simulink model "ProcessNetworkSimulation"  (R2015b)
settings: Solver=VariableStepAuto  StartTime=0.0  StopTime=1000.0  RelTol=1e-3
libraries: simulink x1, simeventslib x1
(part 19 of 21)

== system ProcessNetworkSimulation/Process_48/Process ==
  OUTQueue : FIFOQueue  Capacity=inf
  ProcessQueue : FIFOQueue  Capacity=Inf  StatAverageWait=on  StatAverageQueueLength=on
      settings: OutputPortMap=o2,o3
  ProcessServer : NServer  NumberOfServers=13  ServiceTimeFrom=Signal port t  StatNumberDeparted=on  StatUtilization=on
      settings: OutputPortMap=o0,o5
  ProcessTime : EventBasedRandomNumber  meanExp=0.05  minUnif=1  meanNorm=2  stdNorm=0.2  Seed=7122
  Routing : EventBasedRandomNumber  Distribution=Arbitrary discrete  valueVecDisc=[0,1,2,3,4,5,6,7,8,9,10,11,12,13,14,15,16,17,18,19,20,21,22,23,24,25,26,27,28,29,30,31,32,33,34,35,36,37]  probVecDisc=[0,0.0093,0.0231,0.0139,0.0324,0.0324,0.0231,0.0231,0.0139,0.0459,0.0093,0.0093,0.0093,0.0463,0.0417,0.0417,0.0139,0.037,0.0417,0.0417,0.0324,0.0463,0.0463,0.0324,0.0093,0.0417,0.0093,0.0278,0.0278,0.0139,0.0417,0.0231,0.0093,0.0139,0.0324,0.0417,0.0417,0]  Seed=10339
  read_ProcessTimer : ReadTimer  TimerTag=T_Process_48  StatAverageTimeElapsed=on
      settings: OutputPortMap=o3
  setRouting : SetAttribute  AttributeName=outputFlowNode  AttributeFrom=Signal port  EvaluatedAttributeValue={ []}
  start_ProcessTimer : StartTimer  TimerTag=T_Process_48  TimerStartedOption=Restart
  IN_Job : PMIOPort  Port=1  Side=Left
  OUT_Job : PMIOPort  Port=2  Side=Right
  wires:
  Routing/1 -> setRouting/1
  ProcessTime/1 -> ProcessServer/1
  connections:
  setRouting/LConn1 -- OUTQueue/RConn1
  IN_Job/RConn1 -- start_ProcessTimer/LConn1
  ProcessServer/RConn1 -- read_ProcessTimer/LConn1
  start_ProcessTimer/RConn1 -- ProcessQueue/LConn1
  ProcessQueue/RConn1 -- ProcessServer/LConn1
  read_ProcessTimer/RConn1 -- OUTQueue/LConn1
  OUT_Job/RConn1 -- setRouting/RConn1

== system ProcessNetworkSimulation/Process_49/Process ==
  OUTQueue : FIFOQueue  Capacity=inf
  ProcessQueue : FIFOQueue  Capacity=Inf  StatAverageWait=on  StatAverageQueueLength=on
      settings: OutputPortMap=o2,o3
  ProcessServer : NServer  NumberOfServers=10  ServiceTimeFrom=Signal port t  StatNumberDeparted=on  StatUtilization=on
      settings: OutputPortMap=o0,o5
  ProcessTime : EventBasedRandomNumber  meanExp=0.05  minUnif=1  meanNorm=2  stdNorm=0.2  Seed=13556
  Routing : EventBasedRandomNumber  Distribution=Arbitrary discrete  valueVecDisc=[0,1,2,3,4,5,6,7,8,9,10,11,12,13,14,15,16,17,18,19,20,21,22,23,24,25,26,27,28,29,30,31,32,33,34,35,36,37,38,39,40]  probVecDisc=[0,0.026,0.0104,0.0052,0.026,0.0104,0.0313,0.0104,0.0156,0.0467,0.026,0.0052,0.0104,0.0104,0.0469,0.0156,0.0469,0.0469,0.0104,0.0156,0.0104,0.0365,0.0469,0.0052,0.0156,0.0313,0.0313,0.0365,0.0156,0.0313,0.0365,0.0469,0.0313,0.0156,0.0469,0.0313,0.0156,0.0417,0.0469,0.0104,0]  Seed=16773
  read_ProcessTimer : ReadTimer  TimerTag=T_Process_49  StatAverageTimeElapsed=on
      settings: OutputPortMap=o3
  setRouting : SetAttribute  AttributeName=outputFlowNode  AttributeFrom=Signal port  EvaluatedAttributeValue={ []}
  start_ProcessTimer : StartTimer  TimerTag=T_Process_49  TimerStartedOption=Restart
  IN_Job : PMIOPort  Port=1  Side=Left
  OUT_Job : PMIOPort  Port=2  Side=Right
  wires:
  Routing/1 -> setRouting/1
  ProcessTime/1 -> ProcessServer/1
  connections:
  setRouting/LConn1 -- OUTQueue/RConn1
  IN_Job/RConn1 -- start_ProcessTimer/LConn1
  ProcessServer/RConn1 -- read_ProcessTimer/LConn1
  start_ProcessTimer/RConn1 -- ProcessQueue/LConn1
  ProcessQueue/RConn1 -- ProcessServer/LConn1
  read_ProcessTimer/RConn1 -- OUTQueue/LConn1
  OUT_Job/RConn1 -- setRouting/RConn1

== system ProcessNetworkSimulation/Process_5/Process ==
  OUTQueue : FIFOQueue  Capacity=inf
  ProcessQueue : FIFOQueue  Capacity=Inf  StatAverageWait=on  StatAverageQueueLength=on
      settings: OutputPortMap=o2,o3
  ProcessServer : NServer  NumberOfServers=9  ServiceTimeFrom=Signal port t  StatNumberDeparted=on  StatUtilization=on
      settings: OutputPortMap=o0,o5
  ProcessTime : EventBasedRandomNumber  meanExp=0.05  minUnif=1  meanNorm=2  stdNorm=0.2  Seed=19990
  Routing : EventBasedRandomNumber  Distribution=Arbitrary discrete  valueVecDisc=[0,1,2,3,4,5,6,7,8,9,10,11,12,13,14,15,16,17,18,19,20,21,22,23,24,25,26,27,28,29,30,31,32,33,34,35,36]  probVecDisc=[0,0.0337,0.0112,0.0506,0.0337,0.0056,0.0506,0.0506,0.0112,0.0281,0.0112,0.0281,0.0506,0.0506,0.0112,0.0112,0.0169,0.0393,0.0393,0.0393,0.0112,0.0112,0.0112,0.0112,0.0393,0.0112,0.0506,0.0565,0.0337,0.0281,0.0112,0.0112,0.0112,0.0449,0.0337,0.0506,0]  Seed=23207
  read_ProcessTimer : ReadTimer  TimerTag=T_Process_5  StatAverageTimeElapsed=on
      settings: OutputPortMap=o3
  setRouting : SetAttribute  AttributeName=outputFlowNode  AttributeFrom=Signal port  EvaluatedAttributeValue={ []}
  start_ProcessTimer : StartTimer  TimerTag=T_Process_5  TimerStartedOption=Restart
  IN_Job : PMIOPort  Port=1  Side=Left
  OUT_Job : PMIOPort  Port=2  Side=Right
  wires:
  Routing/1 -> setRouting/1
  ProcessTime/1 -> ProcessServer/1
  connections:
  setRouting/LConn1 -- OUTQueue/RConn1
  IN_Job/RConn1 -- start_ProcessTimer/LConn1
  ProcessServer/RConn1 -- read_ProcessTimer/LConn1
  start_ProcessTimer/RConn1 -- ProcessQueue/LConn1
  ProcessQueue/RConn1 -- ProcessServer/LConn1
  read_ProcessTimer/RConn1 -- OUTQueue/LConn1
  OUT_Job/RConn1 -- setRouting/RConn1

== system ProcessNetworkSimulation/Process_50/Process ==
  OUTQueue : FIFOQueue  Capacity=inf
  ProcessQueue : FIFOQueue  Capacity=Inf  StatAverageWait=on  StatAverageQueueLength=on
      settings: OutputPortMap=o2,o3
  ProcessServer : NServer  NumberOfServers=14  ServiceTimeFrom=Signal port t  StatNumberDeparted=on  StatUtilization=on
      settings: OutputPortMap=o0,o5
  ProcessTime : EventBasedRandomNumber  meanExp=0.05  minUnif=1  meanNorm=2  stdNorm=0.2  Seed=26424
  Routing : EventBasedRandomNumber  Distribution=Arbitrary discrete  valueVecDisc=[0,1,2,3,4,5,6,7,8,9,10,11,12,13,14,15,16,17,18,19,20,21,22,23,24,25,26,27,28,29,30,31,32,33,34,35,36,37,38,39,40,41]  probVecDisc=[0,0.0207,0.0207,0.0331,0.0372,0.0289,0.0124,0.0372,0.0289,0.0207,0.0124,0.0083,0.0248,0.0289,0.0372,0.0083,0.0372,0.0372,0.0083,0.0124,0.0372,0.0083,0.0372,0.0207,0.0289,0.0289,0.0289,0.0207,0.0331,0.0248,0.0372,0.0248,0.0083,0.0408,0.0372,0.0248,0.0372,0.0207,0.0124,0.0083,0.0248,0]  Seed=29641
  read_ProcessTimer : ReadTimer  TimerTag=T_Process_50  StatAverageTimeElapsed=on
      settings: OutputPortMap=o3
  setRouting : SetAttribute  AttributeName=outputFlowNode  AttributeFrom=Signal port  EvaluatedAttributeValue={ []}
  start_ProcessTimer : StartTimer  TimerTag=T_Process_50  TimerStartedOption=Restart
  IN_Job : PMIOPort  Port=1  Side=Left
  OUT_Job : PMIOPort  Port=2  Side=Right
  wires:
  Routing/1 -> setRouting/1
  ProcessTime/1 -> ProcessServer/1
  connections:
  setRouting/LConn1 -- OUTQueue/RConn1
  IN_Job/RConn1 -- start_ProcessTimer/LConn1
  ProcessServer/RConn1 -- read_ProcessTimer/LConn1
  start_ProcessTimer/RConn1 -- ProcessQueue/LConn1
  ProcessQueue/RConn1 -- ProcessServer/LConn1
  read_ProcessTimer/RConn1 -- OUTQueue/LConn1
  OUT_Job/RConn1 -- setRouting/RConn1

== system ProcessNetworkSimulation/Process_51/Process ==
  OUTQueue : FIFOQueue  Capacity=inf
  ProcessQueue : FIFOQueue  Capacity=Inf  StatAverageWait=on  StatAverageQueueLength=on
      settings: OutputPortMap=o2,o3
  ProcessServer : NServer  NumberOfServers=12  ServiceTimeFrom=Signal port t  StatNumberDeparted=on  StatUtilization=on
      settings: OutputPortMap=o0,o5
  ProcessTime : EventBasedRandomNumber  meanExp=0.05  minUnif=1  meanNorm=2  stdNorm=0.2  Seed=32858
  Routing : EventBasedRandomNumber  Distribution=Arbitrary discrete  valueVecDisc=[0,1,2,3,4,5,6,7,8,9,10,11,12,13,14,15,16,17,18,19,20,21,22,23,24,25,26,27,28,29,30,31,32,33,34,35,36,37,38]  probVecDisc=[0,0.0506,0.0462,0.0308,0.0359,0.0308,0.0256,0.0359,0.0308,0.0359,0.0154,0.0359,0.0256,0.0103,0.0256,0.0154,0.0308,0.0103,0.0513,0.0103,0.0359,0.0103,0.0154,0.0103,0.0359,0.0103,0.0154,0.0103,0.0103,0.041,0.0308,0.0103,0.0462,0.0462,0.0359,0.0462,0.0103,0.0256,0]  Seed=36075
  read_ProcessTimer : ReadTimer  TimerTag=T_Process_51  StatAverageTimeElapsed=on
      settings: OutputPortMap=o3
  setRouting : SetAttribute  AttributeName=outputFlowNode  AttributeFrom=Signal port  EvaluatedAttributeValue={ []}
  start_ProcessTimer : StartTimer  TimerTag=T_Process_51  TimerStartedOption=Restart
  IN_Job : PMIOPort  Port=1  Side=Left
  OUT_Job : PMIOPort  Port=2  Side=Right
  wires:
  Routing/1 -> setRouting/1
  ProcessTime/1 -> ProcessServer/1
  connections:
  setRouting/LConn1 -- OUTQueue/RConn1
  IN_Job/RConn1 -- start_ProcessTimer/LConn1
  ProcessServer/RConn1 -- read_ProcessTimer/LConn1
  start_ProcessTimer/RConn1 -- ProcessQueue/LConn1
  ProcessQueue/RConn1 -- ProcessServer/LConn1
  read_ProcessTimer/RConn1 -- OUTQueue/LConn1
  OUT_Job/RConn1 -- setRouting/RConn1

== system ProcessNetworkSimulation/Process_52/Process ==
  OUTQueue : FIFOQueue  Capacity=inf
  ProcessQueue : FIFOQueue  Capacity=Inf  StatAverageWait=on  StatAverageQueueLength=on
      settings: OutputPortMap=o2,o3
  ProcessServer : NServer  NumberOfServers=12  ServiceTimeFrom=Signal port t  StatNumberDeparted=on  StatUtilization=on
      settings: OutputPortMap=o0,o5
  ProcessTime : EventBasedRandomNumber  meanExp=0.05  minUnif=1  meanNorm=2  stdNorm=0.2  Seed=39292
  Routing : EventBasedRandomNumber  Distribution=Arbitrary discrete  valueVecDisc=[0,1,2,3,4,5,6,7,8,9,10,11,12,13,14,15,16,17,18,19,20,21,22,23,24,25,26,27,28,29,30,31,32,33,34,35]  probVecDisc=[0,0.0428,0.0481,0.0107,0.0428,0.0481,0.0107,0.0481,0.0267,0.0481,0.0374,0.0481,0.016,0.0267,0.016,0.0481,0.0053,0.0107,0.0541,0.0321,0.016,0.0321,0.0374,0.0535,0.0267,0.0053,0.016,0.0374,0.0107,0.0481,0.0374,0.0321,0.0053,0.0107,0.0107,0]  Seed=42508
  read_ProcessTimer : ReadTimer  TimerTag=T_Process_52  StatAverageTimeElapsed=on
      settings: OutputPortMap=o3
  setRouting : SetAttribute  AttributeName=outputFlowNode  AttributeFrom=Signal port  EvaluatedAttributeValue={ []}
  start_ProcessTimer : StartTimer  TimerTag=T_Process_52  TimerStartedOption=Restart
  IN_Job : PMIOPort  Port=1  Side=Left
  OUT_Job : PMIOPort  Port=2  Side=Right
  wires:
  Routing/1 -> setRouting/1
  ProcessTime/1 -> ProcessServer/1
  connections:
  setRouting/LConn1 -- OUTQueue/RConn1
  IN_Job/RConn1 -- start_ProcessTimer/LConn1
  ProcessServer/RConn1 -- read_ProcessTimer/LConn1
  start_ProcessTimer/RConn1 -- ProcessQueue/LConn1
  ProcessQueue/RConn1 -- ProcessServer/LConn1
  read_ProcessTimer/RConn1 -- OUTQueue/LConn1
  OUT_Job/RConn1 -- setRouting/RConn1

== system ProcessNetworkSimulation/Process_53/Process ==
  OUTQueue : FIFOQueue  Capacity=inf
  ProcessQueue : FIFOQueue  Capacity=Inf  StatAverageWait=on  StatAverageQueueLength=on
      settings: OutputPortMap=o2,o3
  ProcessServer : NServer  NumberOfServers=10  ServiceTimeFrom=Signal port t  StatNumberDeparted=on  StatUtilization=on
      settings: OutputPortMap=o0,o5
  ProcessTime : EventBasedRandomNumber  meanExp=0.05  minUnif=1  meanNorm=2  stdNorm=0.2  Seed=45725
  Routing : EventBasedRandomNumber  Distribution=Arbitrary discrete  valueVecDisc=[0,1,2,3,4,5,6,7,8,9,10,11,12,13,14,15,16,17,18,19,20,21,22,23,24,25,26,27,28,29,30,31,32,33,34,35,36,37,38,39]  probVecDisc=[0,0.0433,0.024,0.0096,0.0482,0.0096,0.0144,0.0288,0.0433,0.0096,0.0144,0.0337,0.0096,0.024,0.0144,0.0096,0.0288,0.0096,0.0288,0.0096,0.024,0.0433,0.024,0.024,0.0144,0.0433,0.0096,0.0096,0.0433,0.0337,0.0385,0.0096,0.0096,0.0481,0.0433,0.0481,0.0433,0.0433,0.0337,0]  Seed=48942
  read_ProcessTimer : ReadTimer  TimerTag=T_Process_53  StatAverageTimeElapsed=on
      settings: OutputPortMap=o3
  setRouting : SetAttribute  AttributeName=outputFlowNode  AttributeFrom=Signal port  EvaluatedAttributeValue={ []}
  start_ProcessTimer : StartTimer  TimerTag=T_Process_53  TimerStartedOption=Restart
  IN_Job : PMIOPort  Port=1  Side=Left
  OUT_Job : PMIOPort  Port=2  Side=Right
  wires:
  Routing/1 -> setRouting/1
  ProcessTime/1 -> ProcessServer/1
  connections:
  setRouting/LConn1 -- OUTQueue/RConn1
  IN_Job/RConn1 -- start_ProcessTimer/LConn1
  ProcessServer/RConn1 -- read_ProcessTimer/LConn1
  start_ProcessTimer/RConn1 -- ProcessQueue/LConn1
  ProcessQueue/RConn1 -- ProcessServer/LConn1
  read_ProcessTimer/RConn1 -- OUTQueue/LConn1
  OUT_Job/RConn1 -- setRouting/RConn1

== system ProcessNetworkSimulation/Process_54/Process ==
  OUTQueue : FIFOQueue  Capacity=inf
  ProcessQueue : FIFOQueue  Capacity=Inf  StatAverageWait=on  StatAverageQueueLength=on
      settings: OutputPortMap=o2,o3
  ProcessServer : NServer  NumberOfServers=11  ServiceTimeFrom=Signal port t  StatNumberDeparted=on  StatUtilization=on
      settings: OutputPortMap=o0,o5
  ProcessTime : EventBasedRandomNumber  meanExp=0.05  minUnif=1  meanNorm=2  stdNorm=0.2  Seed=52159
  Routing : EventBasedRandomNumber  Distribution=Arbitrary discrete  valueVecDisc=[0,1,2,3,4,5,6,7,8,9,10,11,12,13,14,15,16,17,18,19,20,21,22,23,24,25,26,27,28,29,30,31,32,33,34,35,36,37,38,39,40,41,42,43,44,45,46,47,48,49,50,51]  probVecDisc=[0,0.0174,0.0313,0.0104,0.0278,0.0104,0.0069,0.0035,0.0069,0.0346,0.0208,0.0069,0.0069,0.0347,0.0069,0.0313,0.0278,0.0174,0.0035,0.0243,0.0069,0.0313,0.0069,0.0313,0.0313,0.0208,0.0243,0.0243,0.0243,0.0104,0.0243,0.0243,0.0313,0.0243,0.0174,0.0313,0.0174,0.0069,0.0243,0.0104,0.0208,0.0313,0.0174,0.0313,0.0243,0.0278,0.0208,0.0104,0.0208,0.0104,0.0313,0]  Seed=55376
  read_ProcessTimer : ReadTimer  TimerTag=T_Process_54  StatAverageTimeElapsed=on
      settings: OutputPortMap=o3
  setRouting : SetAttribute  AttributeName=outputFlowNode  AttributeFrom=Signal port  EvaluatedAttributeValue={ []}
  start_ProcessTimer : StartTimer  TimerTag=T_Process_54  TimerStartedOption=Restart
  IN_Job : PMIOPort  Port=1  Side=Left
  OUT_Job : PMIOPort  Port=2  Side=Right
  wires:
  Routing/1 -> setRouting/1
  ProcessTime/1 -> ProcessServer/1
  connections:
  setRouting/LConn1 -- OUTQueue/RConn1
  IN_Job/RConn1 -- start_ProcessTimer/LConn1
  ProcessServer/RConn1 -- read_ProcessTimer/LConn1
  start_ProcessTimer/RConn1 -- ProcessQueue/LConn1
  ProcessQueue/RConn1 -- ProcessServer/LConn1
  read_ProcessTimer/RConn1 -- OUTQueue/LConn1
  OUT_Job/RConn1 -- setRouting/RConn1

== system ProcessNetworkSimulation/Process_55/Process ==
  OUTQueue : FIFOQueue  Capacity=inf
  ProcessQueue : FIFOQueue  Capacity=Inf  StatAverageWait=on  StatAverageQueueLength=on
      settings: OutputPortMap=o2,o3
  ProcessServer : NServer  NumberOfServers=13  ServiceTimeFrom=Signal port t  StatNumberDeparted=on  StatUtilization=on
      settings: OutputPortMap=o0,o5
  ProcessTime : EventBasedRandomNumber  meanExp=0.05  minUnif=1  meanNorm=2  stdNorm=0.2  Seed=58593
  Routing : EventBasedRandomNumber  Distribution=Arbitrary discrete  valueVecDisc=[0,1,2,3,4,5,6,7,8,9,10,11,12,13,14,15,16,17,18,19,20,21,22,23,24,25,26,27,28,29,30,31,32,33,34,35,36,37,38,39,40,41,42,43,44,45,46]  probVecDisc=[0,0.0297,0.0381,0.0339,0.0381,0.0085,0.0381,0.0381,0.0127,0.0085,0.0085,0.0339,0.0254,0.0042,0.0085,0.0085,0.0297,0.0127,0.0085,0.0085,0.0421,0.0297,0.0212,0.0424,0.0212,0.0424,0.0085,0.0381,0.0297,0.0085,0.0297,0.0127,0.0297,0.0042,0.0127,0.0212,0.0254,0.0085,0.0297,0.0254,0.0042,0.0297,0.0085,0.0042,0.0127,0.0424,0.0212]  Seed=61810
  read_ProcessTimer : ReadTimer  TimerTag=T_Process_55  StatAverageTimeElapsed=on
      settings: OutputPortMap=o3
  setRouting : SetAttribute  AttributeName=outputFlowNode  AttributeFrom=Signal port  EvaluatedAttributeValue={ []}
  start_ProcessTimer : StartTimer  TimerTag=T_Process_55  TimerStartedOption=Restart
  IN_Job : PMIOPort  Port=1  Side=Left
  OUT_Job : PMIOPort  Port=2  Side=Right
  wires:
  Routing/1 -> setRouting/1
  ProcessTime/1 -> ProcessServer/1
  connections:
  setRouting/LConn1 -- OUTQueue/RConn1
  IN_Job/RConn1 -- start_ProcessTimer/LConn1
  ProcessServer/RConn1 -- read_ProcessTimer/LConn1
  start_ProcessTimer/RConn1 -- ProcessQueue/LConn1
  ProcessQueue/RConn1 -- ProcessServer/LConn1
  read_ProcessTimer/RConn1 -- OUTQueue/LConn1
  OUT_Job/RConn1 -- setRouting/RConn1

== system ProcessNetworkSimulation/Process_56/Process ==
  OUTQueue : FIFOQueue  Capacity=inf
  ProcessQueue : FIFOQueue  Capacity=Inf  StatAverageWait=on  StatAverageQueueLength=on
      settings: OutputPortMap=o2,o3
  ProcessServer : NServer  NumberOfServers=11  ServiceTimeFrom=Signal port t  StatNumberDeparted=on  StatUtilization=on
      settings: OutputPortMap=o0,o5
  ProcessTime : EventBasedRandomNumber  meanExp=0.05  minUnif=1  meanNorm=2  stdNorm=0.2  Seed=65027
  Routing : EventBasedRandomNumber  Distribution=Arbitrary discrete  valueVecDisc=[0,1,2,3,4,5,6,7,8,9,10,11,12,13,14,15,16,17,18,19,20,21,22,23,24,25,26,27,28,29,30,31,32,33,34,35,36,37,38,39]  probVecDisc=[0,0.0097,0.0242,0.0338,0.0429,0.0097,0.0386,0.0338,0.029,0.0338,0.0145,0.0435,0.029,0.0097,0.0338,0.0242,0.0435,0.0435,0.0435,0.0338,0.0435,0.0242,0.0338,0.0097,0.0435,0.0097,0.0145,0.0145,0.0145,0.029,0.0097,0.0338,0.0435,0.0097,0.0338,0.0097,0.0097,0.0097,0.029,0]  Seed=2708
  read_ProcessTimer : ReadTimer  TimerTag=T_Process_56  StatAverageTimeElapsed=on
      settings: OutputPortMap=o3
  setRouting : SetAttribute  AttributeName=outputFlowNode  AttributeFrom=Signal port  EvaluatedAttributeValue={ []}
  start_ProcessTimer : StartTimer  TimerTag=T_Process_56  TimerStartedOption=Restart
  IN_Job : PMIOPort  Port=1  Side=Left
  OUT_Job : PMIOPort  Port=2  Side=Right
  wires:
  Routing/1 -> setRouting/1
  ProcessTime/1 -> ProcessServer/1
  connections:
  setRouting/LConn1 -- OUTQueue/RConn1
  IN_Job/RConn1 -- start_ProcessTimer/LConn1
  ProcessServer/RConn1 -- read_ProcessTimer/LConn1
  start_ProcessTimer/RConn1 -- ProcessQueue/LConn1
  ProcessQueue/RConn1 -- ProcessServer/LConn1
  read_ProcessTimer/RConn1 -- OUTQueue/LConn1
  OUT_Job/RConn1 -- setRouting/RConn1

== system ProcessNetworkSimulation/Process_57/Process ==
  OUTQueue : FIFOQueue  Capacity=inf
  ProcessQueue : FIFOQueue  Capacity=Inf  StatAverageWait=on  StatAverageQueueLength=on
      settings: OutputPortMap=o2,o3
  ProcessServer : NServer  NumberOfServers=10  ServiceTimeFrom=Signal port t  StatNumberDeparted=on  StatUtilization=on
      settings: OutputPortMap=o0,o5
  ProcessTime : EventBasedRandomNumber  meanExp=0.05  minUnif=1  meanNorm=2  stdNorm=0.2  Seed=5925
  Routing : EventBasedRandomNumber  Distribution=Arbitrary discrete  valueVecDisc=[0,1,2,3,4,5,6,7,8,9,10,11,12,13,14,15,16,17,18,19,20,21,22,23,24,25,26,27,28,29,30,31,32]  probVecDisc=[0,0.0353,0.0118,0.0294,0.0118,0.0471,0.0527,0.0529,0.0471,0.0294,0.0176,0.0529,0.0353,0.0353,0.0353,0.0353,0.0353,0.0294,0.0412,0.0353,0.0412,0.0412,0.0118,0.0294,0.0118,0.0353,0.0412,0.0118,0.0118,0.0353,0.0412,0.0176,0]  Seed=9142
  read_ProcessTimer : ReadTimer  TimerTag=T_Process_57  StatAverageTimeElapsed=on
      settings: OutputPortMap=o3
  setRouting : SetAttribute  AttributeName=outputFlowNode  AttributeFrom=Signal port  EvaluatedAttributeValue={ []}
  start_ProcessTimer : StartTimer  TimerTag=T_Process_57  TimerStartedOption=Restart
  IN_Job : PMIOPort  Port=1  Side=Left
  OUT_Job : PMIOPort  Port=2  Side=Right
  wires:
  Routing/1 -> setRouting/1
  ProcessTime/1 -> ProcessServer/1
  connections:
  setRouting/LConn1 -- OUTQueue/RConn1
  IN_Job/RConn1 -- start_ProcessTimer/LConn1
  ProcessServer/RConn1 -- read_ProcessTimer/LConn1
  start_ProcessTimer/RConn1 -- ProcessQueue/LConn1
  ProcessQueue/RConn1 -- ProcessServer/LConn1
  read_ProcessTimer/RConn1 -- OUTQueue/LConn1
  OUT_Job/RConn1 -- setRouting/RConn1

== system ProcessNetworkSimulation/Process_58/Process ==
  OUTQueue : FIFOQueue  Capacity=inf
  ProcessQueue : FIFOQueue  Capacity=Inf  StatAverageWait=on  StatAverageQueueLength=on
      settings: OutputPortMap=o2,o3
  ProcessServer : NServer  NumberOfServers=15  ServiceTimeFrom=Signal port t  StatNumberDeparted=on  StatUtilization=on
      settings: OutputPortMap=o0,o5
  ProcessTime : EventBasedRandomNumber  meanExp=0.05  minUnif=1  meanNorm=2  stdNorm=0.2  Seed=12359
  Routing : EventBasedRandomNumber  Distribution=Arbitrary discrete  valueVecDisc=[0,1,2,3,4,5,6,7,8,9,10,11,12,13,14,15,16,17,18,19,20,21,22,23,24,25,26,27,28,29,30,31,32,33,34,35,36,37,38,39,40,41,42,43]  probVecDisc=[0,0.0345,0.0307,0.0345,0.0268,0.0192,0.0115,0.0192,0.023,0.0345,0.0077,0.0345,0.0192,0.0115,0.023,0.023,0.023,0.023,0.0038,0.0345,0.023,0.0307,0.0345,0.023,0.0192,0.0192,0.023,0.0115,0.0268,0.0268,0.0038,0.0345,0.0268,0.0345,0.0115,0.0115,0.0378,0.0268,0.0345,0.0307,0.0345,0.0115,0.0268,0]  Seed=15576
  read_ProcessTimer : ReadTimer  TimerTag=T_Process_58  StatAverageTimeElapsed=on
      settings: OutputPortMap=o3
  setRouting : SetAttribute  AttributeName=outputFlowNode  AttributeFrom=Signal port  EvaluatedAttributeValue={ []}
  start_ProcessTimer : StartTimer  TimerTag=T_Process_58  TimerStartedOption=Restart
  IN_Job : PMIOPort  Port=1  Side=Left
  OUT_Job : PMIOPort  Port=2  Side=Right
  wires:
  Routing/1 -> setRouting/1
  ProcessTime/1 -> ProcessServer/1
  connections:
  setRouting/LConn1 -- OUTQueue/RConn1
  IN_Job/RConn1 -- start_ProcessTimer/LConn1
  ProcessServer/RConn1 -- read_ProcessTimer/LConn1
  start_ProcessTimer/RConn1 -- ProcessQueue/LConn1
  ProcessQueue/RConn1 -- ProcessServer/LConn1
  read_ProcessTimer/RConn1 -- OUTQueue/LConn1
  OUT_Job/RConn1 -- setRouting/RConn1

== system ProcessNetworkSimulation/Process_59/Process ==
  OUTQueue : FIFOQueue  Capacity=inf
  ProcessQueue : FIFOQueue  Capacity=Inf  StatAverageWait=on  StatAverageQueueLength=on
      settings: OutputPortMap=o2,o3
  ProcessServer : NServer  NumberOfServers=14  ServiceTimeFrom=Signal port t  StatNumberDeparted=on  StatUtilization=on
      settings: OutputPortMap=o0,o5
  ProcessTime : EventBasedRandomNumber  meanExp=0.05  minUnif=1  meanNorm=2  stdNorm=0.2  Seed=18793
  Routing : EventBasedRandomNumber  Distribution=Arbitrary discrete  valueVecDisc=[0,1,2,3,4,5,6,7,8,9,10,11,12,13,14,15,16,17,18,19,20,21,22,23,24,25,26,27,28,29,30,31,32,33,34,35,36,37,38,39,40,41,42,43,44]  probVecDisc=[0,0.009,0.009,0.009,0.027,0.0045,0.009,0.036,0.0225,0.0315,0.0225,0.0045,0.009,0.009,0.0405,0.0135,0.009,0.0405,0.027,0.0225,0.0315,0.027,0.0315,0.0135,0.0405,0.036,0.027,0.0405,0.027,0.0045,0.0315,0.0315,0.009,0.046,0.0135,0.009,0.0225,0.045,0.009,0.0405,0.009,0.027,0.0405,0.0315,0]  Seed=22010
  read_ProcessTimer : ReadTimer  TimerTag=T_Process_59  StatAverageTimeElapsed=on
      settings: OutputPortMap=o3
  setRouting : SetAttribute  AttributeName=outputFlowNode  AttributeFrom=Signal port  EvaluatedAttributeValue={ []}
  start_ProcessTimer : StartTimer  TimerTag=T_Process_59  TimerStartedOption=Restart
  IN_Job : PMIOPort  Port=1  Side=Left
  OUT_Job : PMIOPort  Port=2  Side=Right
  wires:
  Routing/1 -> setRouting/1
  ProcessTime/1 -> ProcessServer/1
  connections:
  setRouting/LConn1 -- OUTQueue/RConn1
  IN_Job/RConn1 -- start_ProcessTimer/LConn1
  ProcessServer/RConn1 -- read_ProcessTimer/LConn1
  start_ProcessTimer/RConn1 -- ProcessQueue/LConn1
  ProcessQueue/RConn1 -- ProcessServer/LConn1
  read_ProcessTimer/RConn1 -- OUTQueue/LConn1
  OUT_Job/RConn1 -- setRouting/RConn1

== system ProcessNetworkSimulation/Process_6/Process ==
  OUTQueue : FIFOQueue  Capacity=inf
  ProcessQueue : FIFOQueue  Capacity=Inf  StatAverageWait=on  StatAverageQueueLength=on
      settings: OutputPortMap=o2,o3
  ProcessServer : NServer  NumberOfServers=13  ServiceTimeFrom=Signal port t  StatNumberDeparted=on  StatUtilization=on
      settings: OutputPortMap=o0,o5
  ProcessTime : EventBasedRandomNumber  meanExp=0.05  minUnif=1  meanNorm=2  stdNorm=0.2  Seed=25227
  Routing : EventBasedRandomNumber  Distribution=Arbitrary discrete  valueVecDisc=[0,1,2,3,4,5,6,7,8,9,10,11,12,13,14,15,16,17,18,19,20,21,22,23,24,25,26,27,28,29,30,31,32,33,34,35,36,37,38,39]  probVecDisc=[0,0.0096,0.0433,0.0337,0.0433,0.0337,0.0433,0.0337,0.0385,0.0288,0.0433,0.0433,0.024,0.0288,0.0144,0.0096,0.0433,0.0288,0.0433,0.0433,0.0482,0.0144,0.0144,0.0288,0.0433,0.0288,0.0096,0.0096,0.0144,0.0096,0.0096,0.0096,0.0096,0.0385,0.0048,0.0144,0.0096,0.0288,0.0144,0.0096]  Seed=28444
  read_ProcessTimer : ReadTimer  TimerTag=T_Process_6  StatAverageTimeElapsed=on
      settings: OutputPortMap=o3
  setRouting : SetAttribute  AttributeName=outputFlowNode  AttributeFrom=Signal port  EvaluatedAttributeValue={ []}
  start_ProcessTimer : StartTimer  TimerTag=T_Process_6  TimerStartedOption=Restart
  IN_Job : PMIOPort  Port=1  Side=Left
  OUT_Job : PMIOPort  Port=2  Side=Right
  wires:
  Routing/1 -> setRouting/1
  ProcessTime/1 -> ProcessServer/1
  connections:
  setRouting/LConn1 -- OUTQueue/RConn1
  IN_Job/RConn1 -- start_ProcessTimer/LConn1
  ProcessServer/RConn1 -- read_ProcessTimer/LConn1
  start_ProcessTimer/RConn1 -- ProcessQueue/LConn1
  ProcessQueue/RConn1 -- ProcessServer/LConn1
  read_ProcessTimer/RConn1 -- OUTQueue/LConn1
  OUT_Job/RConn1 -- setRouting/RConn1

== system ProcessNetworkSimulation/Process_60/Process ==
  OUTQueue : FIFOQueue  Capacity=inf
  ProcessQueue : FIFOQueue  Capacity=Inf  StatAverageWait=on  StatAverageQueueLength=on
      settings: OutputPortMap=o2,o3
  ProcessServer : NServer  NumberOfServers=11  ServiceTimeFrom=Signal port t  StatNumberDeparted=on  StatUtilization=on
      settings: OutputPortMap=o0,o5
  ProcessTime : EventBasedRandomNumber  meanExp=0.05  minUnif=1  meanNorm=2  stdNorm=0.2  Seed=31661
  Routing : EventBasedRandomNumber  Distribution=Arbitrary discrete  valueVecDisc=[0,1,2,3,4,5,6,7,8,9,10,11,12,13,14,15,16,17,18,19,20,21,22,23,24,25,26,27,28,29,30,31,32,33,34,35,36,37,38,39,40,41]  probVecDisc=[0,0.0424,0.0378,0.0126,0.0378,0.0294,0.0378,0.021,0.0378,0.0336,0.0084,0.0252,0.0378,0.042,0.0042,0.0252,0.021,0.0084,0.0126,0.0294,0.0294,0.0294,0.0336,0.0126,0.021,0.0378,0.0252,0.0084,0.0252,0.0378,0.0084,0.0084,0.0378,0.0378,0.0294,0.0294,0.0084,0.0126,0.0126,0.021,0.0294,0]  Seed=34878
  read_ProcessTimer : ReadTimer  TimerTag=T_Process_60  StatAverageTimeElapsed=on
      settings: OutputPortMap=o3
  setRouting : SetAttribute  AttributeName=outputFlowNode  AttributeFrom=Signal port  EvaluatedAttributeValue={ []}
  start_ProcessTimer : StartTimer  TimerTag=T_Process_60  TimerStartedOption=Restart
  IN_Job : PMIOPort  Port=1  Side=Left
  OUT_Job : PMIOPort  Port=2  Side=Right
  wires:
  Routing/1 -> setRouting/1
  ProcessTime/1 -> ProcessServer/1
  connections:
  setRouting/LConn1 -- OUTQueue/RConn1
  IN_Job/RConn1 -- start_ProcessTimer/LConn1
  ProcessServer/RConn1 -- read_ProcessTimer/LConn1
  start_ProcessTimer/RConn1 -- ProcessQueue/LConn1
  ProcessQueue/RConn1 -- ProcessServer/LConn1
  read_ProcessTimer/RConn1 -- OUTQueue/LConn1
  OUT_Job/RConn1 -- setRouting/RConn1

== system ProcessNetworkSimulation/Process_61/Process ==
  OUTQueue : FIFOQueue  Capacity=inf
  ProcessQueue : FIFOQueue  Capacity=Inf  StatAverageWait=on  StatAverageQueueLength=on
      settings: OutputPortMap=o2,o3
  ProcessServer : NServer  NumberOfServers=14  ServiceTimeFrom=Signal port t  StatNumberDeparted=on  StatUtilization=on
      settings: OutputPortMap=o0,o5
  ProcessTime : EventBasedRandomNumber  meanExp=0.05  minUnif=1  meanNorm=2  stdNorm=0.2  Seed=38095
  Routing : EventBasedRandomNumber  Distribution=Arbitrary discrete  valueVecDisc=[0,1,2,3,4,5,6,7,8,9,10,11,12,13,14,15,16,17,18,19,20,21,22,23,24,25,26,27,28,29,30,31,32,33,34,35,36,37,38,39,40,41,42,43,44]  probVecDisc=[0,0.0039,0.0349,0.038,0.0271,0.0078,0.0349,0.0349,0.0349,0.0349,0.0078,0.0078,0.0116,0.0233,0.0116,0.0271,0.0078,0.0349,0.0349,0.0194,0.0388,0.0078,0.0194,0.0078,0.0233,0.0078,0.0349,0.0349,0.0233,0.0349,0.0271,0.031,0.0078,0.0271,0.0349,0.0194,0.0233,0.0271,0.0271,0.0349,0.0039,0.0194,0.0233,0.0233,0]  Seed=41312
  read_ProcessTimer : ReadTimer  TimerTag=T_Process_61  StatAverageTimeElapsed=on
      settings: OutputPortMap=o3
  setRouting : SetAttribute  AttributeName=outputFlowNode  AttributeFrom=Signal port  EvaluatedAttributeValue={ []}
  start_ProcessTimer : StartTimer  TimerTag=T_Process_61  TimerStartedOption=Restart
  IN_Job : PMIOPort  Port=1  Side=Left
  OUT_Job : PMIOPort  Port=2  Side=Right
  wires:
  Routing/1 -> setRouting/1
  ProcessTime/1 -> ProcessServer/1
  connections:
  setRouting/LConn1 -- OUTQueue/RConn1
  IN_Job/RConn1 -- start_ProcessTimer/LConn1
  ProcessServer/RConn1 -- read_ProcessTimer/LConn1
  start_ProcessTimer/RConn1 -- ProcessQueue/LConn1
  ProcessQueue/RConn1 -- ProcessServer/LConn1
  read_ProcessTimer/RConn1 -- OUTQueue/LConn1
  OUT_Job/RConn1 -- setRouting/RConn1

== system ProcessNetworkSimulation/Process_62/Process ==
  OUTQueue : FIFOQueue  Capacity=inf
  ProcessQueue : FIFOQueue  Capacity=Inf  StatAverageWait=on  StatAverageQueueLength=on
      settings: OutputPortMap=o2,o3
  ProcessServer : NServer  NumberOfServers=9  ServiceTimeFrom=Signal port t  StatNumberDeparted=on  StatUtilization=on
      settings: OutputPortMap=o0,o5
  ProcessTime : EventBasedRandomNumber  meanExp=0.05  minUnif=1  meanNorm=2  stdNorm=0.2  Seed=44529
  Routing : EventBasedRandomNumber  Distribution=Arbitrary discrete  valueVecDisc=[0,1,2,3,4,5,6,7,8,9,10,11,12,13,14,15,16,17,18,19,20,21,22,23,24,25,26,27,28,29,30,31,32,33,34,35,36,37,38,39,40,41]  probVecDisc=[0,0.0372,0.0106,0.0479,0.0319,0.0106,0.016,0.0106,0.0053,0.0319,0.0536,0.0266,0.0106,0.0372,0.0106,0.0266,0.0053,0.0479,0.0319,0.0106,0.016,0.0266,0.0106,0.0479,0.0106,0.0266,0.016,0.0106,0.0372,0.0479,0.0372,0.0106,0.016,0.0266,0.0266,0.0266,0.0319,0.0372,0.0106,0.0372,0.0266,0]  Seed=47746
  read_ProcessTimer : ReadTimer  TimerTag=T_Process_62  StatAverageTimeElapsed=on
      settings: OutputPortMap=o3
  setRouting : SetAttribute  AttributeName=outputFlowNode  AttributeFrom=Signal port  EvaluatedAttributeValue={ []}
  start_ProcessTimer : StartTimer  TimerTag=T_Process_62  TimerStartedOption=Restart
  IN_Job : PMIOPort  Port=1  Side=Left
  OUT_Job : PMIOPort  Port=2  Side=Right
  wires:
  Routing/1 -> setRouting/1
  ProcessTime/1 -> ProcessServer/1
  connections:
  setRouting/LConn1 -- OUTQueue/RConn1
  IN_Job/RConn1 -- start_ProcessTimer/LConn1
  ProcessServer/RConn1 -- read_ProcessTimer/LConn1
  start_ProcessTimer/RConn1 -- ProcessQueue/LConn1
  ProcessQueue/RConn1 -- ProcessServer/LConn1
  read_ProcessTimer/RConn1 -- OUTQueue/LConn1
  OUT_Job/RConn1 -- setRouting/RConn1

== system ProcessNetworkSimulation/Process_63/Process ==
  OUTQueue : FIFOQueue  Capacity=inf
  ProcessQueue : FIFOQueue  Capacity=Inf  StatAverageWait=on  StatAverageQueueLength=on
      settings: OutputPortMap=o2,o3
  ProcessServer : NServer  NumberOfServers=13  ServiceTimeFrom=Signal port t  StatNumberDeparted=on  StatUtilization=on
      settings: OutputPortMap=o0,o5
  ProcessTime : EventBasedRandomNumber  meanExp=0.05  minUnif=1  meanNorm=2  stdNorm=0.2  Seed=50963
  Routing : EventBasedRandomNumber  Distribution=Arbitrary discrete  valueVecDisc=[0,1,2,3,4,5,6,7,8,9,10,11,12,13,14,15,16,17,18,19,20,21,22,23,24,25,26,27,28,29,30,31,32,33,34,35,36,37,38,39,40,41,42]  probVecDisc=[0,0.0091,0.0273,0.0318,0.0273,0.0318,0.0091,0.0318,0.0227,0.0273,0.0273,0.0273,0.0409,0.0409,0.0091,0.0409,0.0091,0.0318,0.0318,0.0091,0.0136,0.0227,0.0318,0.0273,0.0273,0.0273,0.0409,0.0409,0.0091,0.0409,0.0091,0.0273,0.0318,0.0227,0.0091,0.0091,0.0091,0.0273,0.0318,0.0045,0.0409,0.0091,0]  Seed=54180
  read_ProcessTimer : ReadTimer  TimerTag=T_Process_63  StatAverageTimeElapsed=on
      settings: OutputPortMap=o3
  setRouting : SetAttribute  AttributeName=outputFlowNode  AttributeFrom=Signal port  EvaluatedAttributeValue={ []}
  start_ProcessTimer : StartTimer  TimerTag=T_Process_63  TimerStartedOption=Restart
  IN_Job : PMIOPort  Port=1  Side=Left
  OUT_Job : PMIOPort  Port=2  Side=Right
  wires:
  Routing/1 -> setRouting/1
  ProcessTime/1 -> ProcessServer/1
  connections:
  setRouting/LConn1 -- OUTQueue/RConn1
  IN_Job/RConn1 -- start_ProcessTimer/LConn1
  ProcessServer/RConn1 -- read_ProcessTimer/LConn1
  start_ProcessTimer/RConn1 -- ProcessQueue/LConn1
  ProcessQueue/RConn1 -- ProcessServer/LConn1
  read_ProcessTimer/RConn1 -- OUTQueue/LConn1
  OUT_Job/RConn1 -- setRouting/RConn1

== system ProcessNetworkSimulation/Process_64/Process ==
  OUTQueue : FIFOQueue  Capacity=inf
  ProcessQueue : FIFOQueue  Capacity=Inf  StatAverageWait=on  StatAverageQueueLength=on
      settings: OutputPortMap=o2,o3
  ProcessServer : NServer  NumberOfServers=10  ServiceTimeFrom=Signal port t  StatNumberDeparted=on  StatUtilization=on
      settings: OutputPortMap=o0,o5
  ProcessTime : EventBasedRandomNumber  meanExp=0.05  minUnif=1  meanNorm=2  stdNorm=0.2  Seed=57397
  Routing : EventBasedRandomNumber  Distribution=Arbitrary discrete  valueVecDisc=[0,1,2,3,4,5,6,7,8,9,10,11,12,13,14,15,16,17,18,19,20,21,22,23,24,25,26,27,28,29,30,31,32,33,34,35,36]  probVecDisc=[0,0.0357,0.0357,0.0357,0.0357,0.0119,0.0357,0.0179,0.0417,0.0532,0.0417,0.0179,0.0476,0.0119,0.0476,0.0298,0.0357,0.0417,0.0179,0.0298,0.0119,0.0119,0.0119,0.006,0.0357,0.0357,0.0417,0.006,0.0119,0.0357,0.0536,0.0357,0.0417,0.0179,0.0119,0.006,0]  Seed=60614
  read_ProcessTimer : ReadTimer  TimerTag=T_Process_64  StatAverageTimeElapsed=on
      settings: OutputPortMap=o3
  setRouting : SetAttribute  AttributeName=outputFlowNode  AttributeFrom=Signal port  EvaluatedAttributeValue={ []}
  start_ProcessTimer : StartTimer  TimerTag=T_Process_64  TimerStartedOption=Restart
  IN_Job : PMIOPort  Port=1  Side=Left
  OUT_Job : PMIOPort  Port=2  Side=Right
  wires:
  Routing/1 -> setRouting/1
  ProcessTime/1 -> ProcessServer/1
  connections:
  setRouting/LConn1 -- OUTQueue/RConn1
  IN_Job/RConn1 -- start_ProcessTimer/LConn1
  ProcessServer/RConn1 -- read_ProcessTimer/LConn1
  start_ProcessTimer/RConn1 -- ProcessQueue/LConn1
  ProcessQueue/RConn1 -- ProcessServer/LConn1
  read_ProcessTimer/RConn1 -- OUTQueue/LConn1
  OUT_Job/RConn1 -- setRouting/RConn1

== system ProcessNetworkSimulation/Process_65/Process ==
  OUTQueue : FIFOQueue  Capacity=inf
  ProcessQueue : FIFOQueue  Capacity=Inf  StatAverageWait=on  StatAverageQueueLength=on
      settings: OutputPortMap=o2,o3
  ProcessServer : NServer  NumberOfServers=10  ServiceTimeFrom=Signal port t  StatNumberDeparted=on  StatUtilization=on
      settings: OutputPortMap=o0,o5
  ProcessTime : EventBasedRandomNumber  meanExp=0.05  minUnif=1  meanNorm=2  stdNorm=0.2  Seed=63831
  Routing : EventBasedRandomNumber  Distribution=Arbitrary discrete  valueVecDisc=[0,1,2,3,4,5,6,7,8,9,10,11,12,13,14,15,16,17,18,19,20,21,22,23,24,25,26,27,28,29,30,31,32,33,34,35,36,37]  probVecDisc=[0,0.0057,0.0519,0.0114,0.0457,0.0343,0.0514,0.04,0.0114,0.0514,0.0114,0.0114,0.0171,0.0171,0.0286,0.0057,0.04,0.0171,0.04,0.0114,0.0457,0.0114,0.0114,0.04,0.04,0.0343,0.04,0.04,0.0286,0.0114,0.0171,0.04,0.0286,0.0114,0.0114,0.0343,0.0514,0]  Seed=1512
  read_ProcessTimer : ReadTimer  TimerTag=T_Process_65  StatAverageTimeElapsed=on
      settings: OutputPortMap=o3
  setRouting : SetAttribute  AttributeName=outputFlowNode  AttributeFrom=Signal port  EvaluatedAttributeValue={ []}
  start_ProcessTimer : StartTimer  TimerTag=T_Process_65  TimerStartedOption=Restart
  IN_Job : PMIOPort  Port=1  Side=Left
  OUT_Job : PMIOPort  Port=2  Side=Right
  wires:
  Routing/1 -> setRouting/1
  ProcessTime/1 -> ProcessServer/1
  connections:
  setRouting/LConn1 -- OUTQueue/RConn1
  IN_Job/RConn1 -- start_ProcessTimer/LConn1
  ProcessServer/RConn1 -- read_ProcessTimer/LConn1
  start_ProcessTimer/RConn1 -- ProcessQueue/LConn1
  ProcessQueue/RConn1 -- ProcessServer/LConn1
  read_ProcessTimer/RConn1 -- OUTQueue/LConn1
  OUT_Job/RConn1 -- setRouting/RConn1

== system ProcessNetworkSimulation/Process_66/Process ==
  OUTQueue : FIFOQueue  Capacity=inf
  ProcessQueue : FIFOQueue  Capacity=Inf  StatAverageWait=on  StatAverageQueueLength=on
      settings: OutputPortMap=o2,o3
  ProcessServer : NServer  NumberOfServers=13  ServiceTimeFrom=Signal port t  StatNumberDeparted=on  StatUtilization=on
      settings: OutputPortMap=o0,o5
  ProcessTime : EventBasedRandomNumber  meanExp=0.05  minUnif=1  meanNorm=2  stdNorm=0.2  Seed=4729
  Routing : EventBasedRandomNumber  Distribution=Arbitrary discrete  valueVecDisc=[0,1,2,3,4,5,6,7,8,9,10,11,12,13,14,15,16,17,18,19,20,21,22,23,24,25,26,27,28,29,30,31,32,33,34,35,36,37,38,39,40,41,42]  probVecDisc=[0,0.0462,0.0282,0.0094,0.0469,0.0235,0.0282,0.0094,0.0094,0.0376,0.0094,0.0329,0.0094,0.0282,0.0141,0.0235,0.0469,0.0235,0.0423,0.0282,0.0094,0.0282,0.0141,0.0329,0.0282,0.0376,0.0141,0.0423,0.0094,0.0047,0.0423,0.0047,0.0235,0.0141,0.0329,0.0329,0.0141,0.0376,0.0094,0.0094,0.0141,0.0469,0]  Seed=7946
  read_ProcessTimer : ReadTimer  TimerTag=T_Process_66  StatAverageTimeElapsed=on
      settings: OutputPortMap=o3
  setRouting : SetAttribute  AttributeName=outputFlowNode  AttributeFrom=Signal port  EvaluatedAttributeValue={ []}
  start_ProcessTimer : StartTimer  TimerTag=T_Process_66  TimerStartedOption=Restart
  IN_Job : PMIOPort  Port=1  Side=Left
  OUT_Job : PMIOPort  Port=2  Side=Right
  wires:
  Routing/1 -> setRouting/1
  ProcessTime/1 -> ProcessServer/1
  connections:
  setRouting/LConn1 -- OUTQueue/RConn1
  IN_Job/RConn1 -- start_ProcessTimer/LConn1
  ProcessServer/RConn1 -- read_ProcessTimer/LConn1
  start_ProcessTimer/RConn1 -- ProcessQueue/LConn1
  ProcessQueue/RConn1 -- ProcessServer/LConn1
  read_ProcessTimer/RConn1 -- OUTQueue/LConn1
  OUT_Job/RConn1 -- setRouting/RConn1

== system ProcessNetworkSimulation/Process_67/Process ==
  OUTQueue : FIFOQueue  Capacity=inf
  ProcessQueue : FIFOQueue  Capacity=Inf  StatAverageWait=on  StatAverageQueueLength=on
      settings: OutputPortMap=o2,o3
  ProcessServer : NServer  NumberOfServers=9  ServiceTimeFrom=Signal port t  StatNumberDeparted=on  StatUtilization=on
      settings: OutputPortMap=o0,o5
  ProcessTime : EventBasedRandomNumber  meanExp=0.05  minUnif=1  meanNorm=2  stdNorm=0.2  Seed=11163
  Routing : EventBasedRandomNumber  Distribution=Arbitrary discrete  valueVecDisc=[0,1,2,3,4,5,6,7,8,9,10,11,12,13,14,15,16,17,18,19,20,21,22,23,24,25,26,27,28,29,30,31,32,33,34,35]  probVecDisc=[0,0.0053,0.016,0.0266,0.0106,0.0106,0.0106,0.0053,0.0372,0.0053,0.0266,0.0106,0.048,0.0426,0.0372,0.0372,0.0372,0.0479,0.0372,0.0479,0.0479,0.0479,0.0266,0.0106,0.0479,0.0479,0.0106,0.0266,0.0319,0.0372,0.0319,0.0479,0.0426,0.0266,0.016,0]  Seed=14380
  read_ProcessTimer : ReadTimer  TimerTag=T_Process_67  StatAverageTimeElapsed=on
      settings: OutputPortMap=o3
  setRouting : SetAttribute  AttributeName=outputFlowNode  AttributeFrom=Signal port  EvaluatedAttributeValue={ []}
  start_ProcessTimer : StartTimer  TimerTag=T_Process_67  TimerStartedOption=Restart
  IN_Job : PMIOPort  Port=1  Side=Left
  OUT_Job : PMIOPort  Port=2  Side=Right
  wires:
  Routing/1 -> setRouting/1
  ProcessTime/1 -> ProcessServer/1
  connections:
  setRouting/LConn1 -- OUTQueue/RConn1
  IN_Job/RConn1 -- start_ProcessTimer/LConn1
  ProcessServer/RConn1 -- read_ProcessTimer/LConn1
  start_ProcessTimer/RConn1 -- ProcessQueue/LConn1
  ProcessQueue/RConn1 -- ProcessServer/LConn1
  read_ProcessTimer/RConn1 -- OUTQueue/LConn1
  OUT_Job/RConn1 -- setRouting/RConn1

== system ProcessNetworkSimulation/Process_68/Process ==
  OUTQueue : FIFOQueue  Capacity=inf
  ProcessQueue : FIFOQueue  Capacity=Inf  StatAverageWait=on  StatAverageQueueLength=on
      settings: OutputPortMap=o2,o3
  ProcessServer : NServer  NumberOfServers=11  ServiceTimeFrom=Signal port t  StatNumberDeparted=on  StatUtilization=on
      settings: OutputPortMap=o0,o5
  ProcessTime : EventBasedRandomNumber  meanExp=0.05  minUnif=1  meanNorm=2  stdNorm=0.2  Seed=17597
  Routing : EventBasedRandomNumber  Distribution=Arbitrary discrete  valueVecDisc=[0,1,2,3,4,5,6,7,8,9,10,11,12,13,14,15,16,17,18,19,20,21,22,23,24,25,26,27,28,29,30,31,32,33,34,35,36,37,38,39,40,41,42,43]  probVecDisc=[0,0.0446,0.0251,0.0452,0.0452,0.0101,0.0101,0.0452,0.005,0.0251,0.005,0.0302,0.0302,0.0101,0.0251,0.0302,0.0151,0.0101,0.0302,0.0452,0.0302,0.0251,0.0302,0.0251,0.0101,0.0352,0.0402,0.0101,0.0101,0.0352,0.0251,0.0101,0.005,0.0251,0.0151,0.0452,0.0101,0.0101,0.0402,0.0101,0.0452,0.0101,0.0101,0]  Seed=20814
  read_ProcessTimer : ReadTimer  TimerTag=T_Process_68  StatAverageTimeElapsed=on
      settings: OutputPortMap=o3
  setRouting : SetAttribute  AttributeName=outputFlowNode  AttributeFrom=Signal port  EvaluatedAttributeValue={ []}
  start_ProcessTimer : StartTimer  TimerTag=T_Process_68  TimerStartedOption=Restart
  IN_Job : PMIOPort  Port=1  Side=Left
  OUT_Job : PMIOPort  Port=2  Side=Right
  wires:
  Routing/1 -> setRouting/1
  ProcessTime/1 -> ProcessServer/1
  connections:
  setRouting/LConn1 -- OUTQueue/RConn1
  IN_Job/RConn1 -- start_ProcessTimer/LConn1
  ProcessServer/RConn1 -- read_ProcessTimer/LConn1
  start_ProcessTimer/RConn1 -- ProcessQueue/LConn1
  ProcessQueue/RConn1 -- ProcessServer/LConn1
  read_ProcessTimer/RConn1 -- OUTQueue/LConn1
  OUT_Job/RConn1 -- setRouting/RConn1

== system ProcessNetworkSimulation/Process_69/Process ==
  OUTQueue : FIFOQueue  Capacity=inf
  ProcessQueue : FIFOQueue  Capacity=Inf  StatAverageWait=on  StatAverageQueueLength=on
      settings: OutputPortMap=o2,o3
  ProcessServer : NServer  NumberOfServers=11  ServiceTimeFrom=Signal port t  StatNumberDeparted=on  StatUtilization=on
      settings: OutputPortMap=o0,o5
  ProcessTime : EventBasedRandomNumber  meanExp=0.05  minUnif=1  meanNorm=2  stdNorm=0.2  Seed=24031
  Routing : EventBasedRandomNumber  Distribution=Arbitrary discrete  valueVecDisc=[0,1,2,3,4,5,6,7,8,9,10,11,12,13,14,15,16,17,18,19,20,21,22,23,24,25,26,27,28,29,30,31,32,33,34,35,36,37,38,39,40,41]  probVecDisc=[0,0.008,0.032,0.036,0.04,0.028,0.028,0.028,0.02,0.008,0.036,0.008,0.036,0.036,0.012,0.032,0.032,0.028,0.024,0.008,0.036,0.008,0.036,0.02,0.036,0.032,0.036,0.008,0.04,0.028,0.02,0.008,0.02,0.036,0.02,0.008,0.02,0.04,0.028,0.008,0.008,0.024]  Seed=27248
  read_ProcessTimer : ReadTimer  TimerTag=T_Process_69  StatAverageTimeElapsed=on
      settings: OutputPortMap=o3
  setRouting : SetAttribute  AttributeName=outputFlowNode  AttributeFrom=Signal port  EvaluatedAttributeValue={ []}
  start_ProcessTimer : StartTimer  TimerTag=T_Process_69  TimerStartedOption=Restart
  IN_Job : PMIOPort  Port=1  Side=Left
  OUT_Job : PMIOPort  Port=2  Side=Right
  wires:
  Routing/1 -> setRouting/1
  ProcessTime/1 -> ProcessServer/1
  connections:
  setRouting/LConn1 -- OUTQueue/RConn1
  IN_Job/RConn1 -- start_ProcessTimer/LConn1
  ProcessServer/RConn1 -- read_ProcessTimer/LConn1
  start_ProcessTimer/RConn1 -- ProcessQueue/LConn1
  ProcessQueue/RConn1 -- ProcessServer/LConn1
  read_ProcessTimer/RConn1 -- OUTQueue/LConn1
  OUT_Job/RConn1 -- setRouting/RConn1

== system ProcessNetworkSimulation/Process_7/Process ==
  OUTQueue : FIFOQueue  Capacity=inf
  ProcessQueue : FIFOQueue  Capacity=Inf  StatAverageWait=on  StatAverageQueueLength=on
      settings: OutputPortMap=o2,o3
  ProcessServer : NServer  NumberOfServers=13  ServiceTimeFrom=Signal port t  StatNumberDeparted=on  StatUtilization=on
      settings: OutputPortMap=o0,o5
  ProcessTime : EventBasedRandomNumber  meanExp=0.05  minUnif=1  meanNorm=2  stdNorm=0.2  Seed=30465
  Routing : EventBasedRandomNumber  Distribution=Arbitrary discrete  valueVecDisc=[0,1,2,3,4,5,6,7,8,9,10,11,12,13,14,15,16,17,18,19,20,21,22,23,24,25,26,27,28,29,30,31,32,33,34,35,36,37,38,39,40,41,42]  probVecDisc=[0,0.0129,0.0388,0.0086,0.0129,0.0388,0.0216,0.0388,0.0129,0.0259,0.0129,0.0388,0.0302,0.0302,0.0388,0.0086,0.0086,0.0388,0.0259,0.0302,0.0216,0.0216,0.0086,0.0388,0.0129,0.0086,0.0345,0.0043,0.0302,0.0216,0.0259,0.0388,0.0427,0.0086,0.0302,0.0086,0.0216,0.0345,0.0259,0.0259,0.0388,0.0216,0]  Seed=33682
  read_ProcessTimer : ReadTimer  TimerTag=T_Process_7  StatAverageTimeElapsed=on
      settings: OutputPortMap=o3
  setRouting : SetAttribute  AttributeName=outputFlowNode  AttributeFrom=Signal port  EvaluatedAttributeValue={ []}
  start_ProcessTimer : StartTimer  TimerTag=T_Process_7  TimerStartedOption=Restart
  IN_Job : PMIOPort  Port=1  Side=Left
  OUT_Job : PMIOPort  Port=2  Side=Right
  wires:
  Routing/1 -> setRouting/1
  ProcessTime/1 -> ProcessServer/1
  connections:
  setRouting/LConn1 -- OUTQueue/RConn1
  IN_Job/RConn1 -- start_ProcessTimer/LConn1
  ProcessServer/RConn1 -- read_ProcessTimer/LConn1
  start_ProcessTimer/RConn1 -- ProcessQueue/LConn1
  ProcessQueue/RConn1 -- ProcessServer/LConn1
  read_ProcessTimer/RConn1 -- OUTQueue/LConn1
  OUT_Job/RConn1 -- setRouting/RConn1

== system ProcessNetworkSimulation/Process_70/Process ==
  OUTQueue : FIFOQueue  Capacity=inf
  ProcessQueue : FIFOQueue  Capacity=Inf  StatAverageWait=on  StatAverageQueueLength=on
      settings: OutputPortMap=o2,o3
  ProcessServer : NServer  NumberOfServers=10  ServiceTimeFrom=Signal port t  StatNumberDeparted=on  StatUtilization=on
      settings: OutputPortMap=o0,o5
  ProcessTime : EventBasedRandomNumber  meanExp=0.05  minUnif=1  meanNorm=2  stdNorm=0.2  Seed=36899
  Routing : EventBasedRandomNumber  Distribution=Arbitrary discrete  valueVecDisc=[0,1,2,3,4,5,6,7,8,9,10,11,12,13,14,15,16,17,18,19,20,21,22,23,24,25,26,27,28,29,30,31,32,33,34,35,36,37]  probVecDisc=[0,0.0348,0.01,0.0448,0.0249,0.0487,0.01,0.0299,0.0448,0.01,0.0448,0.0398,0.0398,0.005,0.0448,0.0249,0.0498,0.0299,0.01,0.0448,0.0299,0.0299,0.0249,0.01,0.0249,0.0299,0.01,0.0299,0.01,0.0448,0.0348,0.01,0.01,0.0348,0.01,0.0498,0.0149,0]  Seed=40116
  read_ProcessTimer : ReadTimer  TimerTag=T_Process_70  StatAverageTimeElapsed=on
      settings: OutputPortMap=o3
  setRouting : SetAttribute  AttributeName=outputFlowNode  AttributeFrom=Signal port  EvaluatedAttributeValue={ []}
  start_ProcessTimer : StartTimer  TimerTag=T_Process_70  TimerStartedOption=Restart
  IN_Job : PMIOPort  Port=1  Side=Left
  OUT_Job : PMIOPort  Port=2  Side=Right
  wires:
  Routing/1 -> setRouting/1
  ProcessTime/1 -> ProcessServer/1
  connections:
  setRouting/LConn1 -- OUTQueue/RConn1
  IN_Job/RConn1 -- start_ProcessTimer/LConn1
  ProcessServer/RConn1 -- read_ProcessTimer/LConn1
  start_ProcessTimer/RConn1 -- ProcessQueue/LConn1
  ProcessQueue/RConn1 -- ProcessServer/LConn1
  read_ProcessTimer/RConn1 -- OUTQueue/LConn1
  OUT_Job/RConn1 -- setRouting/RConn1

== system ProcessNetworkSimulation/Process_71/Process ==
  OUTQueue : FIFOQueue  Capacity=inf
  ProcessQueue : FIFOQueue  Capacity=Inf  StatAverageWait=on  StatAverageQueueLength=on
      settings: OutputPortMap=o2,o3
  ProcessServer : NServer  NumberOfServers=9  ServiceTimeFrom=Signal port t  StatNumberDeparted=on  StatUtilization=on
      settings: OutputPortMap=o0,o5
  ProcessTime : EventBasedRandomNumber  meanExp=0.05  minUnif=1  meanNorm=2  stdNorm=0.2  Seed=43333
  Routing : EventBasedRandomNumber  Distribution=Arbitrary discrete  valueVecDisc=[0,1,2,3,4,5,6,7,8,9,10,11,12,13,14,15,16,17,18,19,20,21,22,23,24,25,26,27,28,29,30,31,32,33,34,35,36,37,38,39,40,41,42]  probVecDisc=[0,0.0102,0.0355,0.0406,0.0152,0.0051,0.0254,0.0305,0.0254,0.0102,0.0102,0.0355,0.0355,0.0102,0.0102,0.0305,0.0355,0.0102,0.0102,0.0406,0.0102,0.0254,0.0305,0.0457,0.0355,0.0051,0.0102,0.0355,0.05,0.0102,0.0305,0.0457,0.0102,0.0254,0.0254,0.0102,0.0457,0.0457,0.0051,0.0102,0.0254,0.0355,0]  Seed=46550
  read_ProcessTimer : ReadTimer  TimerTag=T_Process_71  StatAverageTimeElapsed=on
      settings: OutputPortMap=o3
  setRouting : SetAttribute  AttributeName=outputFlowNode  AttributeFrom=Signal port  EvaluatedAttributeValue={ []}
  start_ProcessTimer : StartTimer  TimerTag=T_Process_71  TimerStartedOption=Restart
  IN_Job : PMIOPort  Port=1  Side=Left
  OUT_Job : PMIOPort  Port=2  Side=Right
  wires:
  Routing/1 -> setRouting/1
  ProcessTime/1 -> ProcessServer/1
  connections:
  setRouting/LConn1 -- OUTQueue/RConn1
  IN_Job/RConn1 -- start_ProcessTimer/LConn1
  ProcessServer/RConn1 -- read_ProcessTimer/LConn1
  start_ProcessTimer/RConn1 -- ProcessQueue/LConn1
  ProcessQueue/RConn1 -- ProcessServer/LConn1
  read_ProcessTimer/RConn1 -- OUTQueue/LConn1
  OUT_Job/RConn1 -- setRouting/RConn1

== system ProcessNetworkSimulation/Process_72/Process ==
  OUTQueue : FIFOQueue  Capacity=inf
  ProcessQueue : FIFOQueue  Capacity=Inf  StatAverageWait=on  StatAverageQueueLength=on
      settings: OutputPortMap=o2,o3
  ProcessServer : NServer  NumberOfServers=8  ServiceTimeFrom=Signal port t  StatNumberDeparted=on  StatUtilization=on
      settings: OutputPortMap=o0,o5
  ProcessTime : EventBasedRandomNumber  meanExp=0.05  minUnif=1  meanNorm=2  stdNorm=0.2  Seed=49767
  Routing : EventBasedRandomNumber  Distribution=Arbitrary discrete  valueVecDisc=[0,1,2,3,4,5,6,7,8,9,10,11,12,13,14,15,16,17,18,19,20,21,22,23,24,25,26,27,28,29,30,31,32,33,34,35]  probVecDisc=[0,0.0443,0.0127,0.0127,0.0127,0.057,0.057,0.0443,0.019,0.0127,0.0316,0.019,0.0443,0.038,0.0443,0.019,0.0127,0.0443,0.0506,0.0443,0.019,0.063,0.0316,0.0127,0.0316,0.019,0.019,0.0127,0.0127,0.0316,0.0063,0.0127,0.038,0.038,0.0316,0]  Seed=52984
  read_ProcessTimer : ReadTimer  TimerTag=T_Process_72  StatAverageTimeElapsed=on
      settings: OutputPortMap=o3
  setRouting : SetAttribute  AttributeName=outputFlowNode  AttributeFrom=Signal port  EvaluatedAttributeValue={ []}
  start_ProcessTimer : StartTimer  TimerTag=T_Process_72  TimerStartedOption=Restart
  IN_Job : PMIOPort  Port=1  Side=Left
  OUT_Job : PMIOPort  Port=2  Side=Right
  wires:
  Routing/1 -> setRouting/1
  ProcessTime/1 -> ProcessServer/1
  connections:
  setRouting/LConn1 -- OUTQueue/RConn1
  IN_Job/RConn1 -- start_ProcessTimer/LConn1
  ProcessServer/RConn1 -- read_ProcessTimer/LConn1
  start_ProcessTimer/RConn1 -- ProcessQueue/LConn1
  ProcessQueue/RConn1 -- ProcessServer/LConn1
  read_ProcessTimer/RConn1 -- OUTQueue/LConn1
  OUT_Job/RConn1 -- setRouting/RConn1
